simulink model "IMUControl"  (R2019b)
settings: Solver=FixedStepAuto  StartTime=0.0  StopTime=10.0  RelTol=1e-3
libraries: androidsensorlib x4, androiduilib x2, androidadvancedlib x1
settings Model: Creator=The MathWorks, Inc.  LastModifiedBy=Bilal
settings OptimizationCC: EnhancedBackFolding=on  PassReuseOutputArgsThreshold=0  MaxStackSize=64  OptimizeBlockOrder=speed  DifferentSizesBufferReuse=on  OptimizationCustomize=off
settings DebuggingCC: ParameterTunabilityLossMsg=error  ArithmeticOperatorsInVariantConditions=warning
settings HardwareCC: ProdBitPerPointer=32  ProdBitPerSizeT=32  ProdBitPerPtrDiffT=32  ProdLargestAtomicInteger=Long  ProdLargestAtomicFloat=Double  ProdWordSize=32  ProdHWDeviceType=ARM Compatible->ARM Cortex  UseEmbeddedCoderFeatures=off  UseSimulinkCoderFeatures=off
settings SFSimCC: MATLABDynamicMemAlloc=off  CustomCodeUndefinedFunction=UseInterfaceOnly
settings RTWCC: SystemTargetFile=ert.tlc  HardwareBoard=Android Device  TLCOptions="-aInlineSetEventsForThisBaseRateFcn=TLC_FALSE -aSuppressMultiTaskScheduler=TLC_FALSE  -aRateBasedStepFcn=0"  TemplateMakefile=ert_default_tmf  GenerateReport=on  RTWVerbose=off  Toolchain=Android SDK/NDK Tools  LaunchReport=on
settings CodeAppCC: ForceParamTrailComments=on  OperatorAnnotations=on
settings ERTTargetCC: ERTCustomFileBanners=off  SupportContinuousTime=on  SupportNonInlinedSFcns=on  RemoveResetFunc=off  ModelStepFunctionPrototypeControlCompliant=off

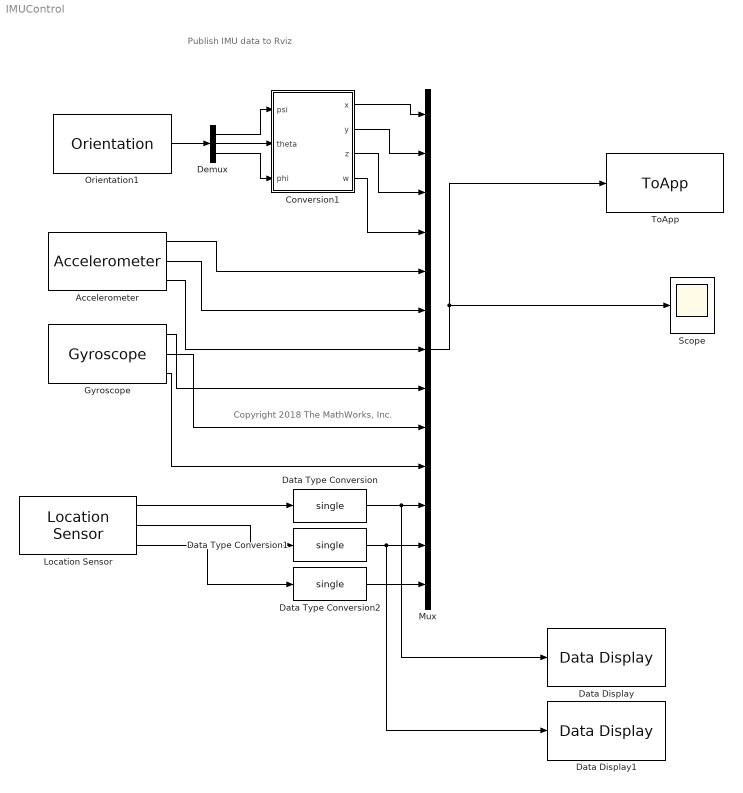
== system IMUControl ==
  note: Copyright 2018 The MathWorks, Inc.
  note: Publish IMU data to Rviz
  Accelerometer : androidsensorlib/Accelerometer  OutputVector=off  SampleTime=0.1  BlockPlatform=Android
      settings: SourceProductName=Simulink Support Package for Android Devices  SourceProductBaseCode=ANDROID
  Conversion1 : MATLAB Function  TreatAsAtomicUnit=on
  Data Display : androiduilib/Data Display  Format=Float  Precision=6  SimulateUsing=Code generation  blockPlatform=Android
      settings: SourceProductName=Simulink Support Package for Android Devices  SourceProductBaseCode=ANDROID
  Data Display1 : androiduilib/Data Display  Format=Float  Precision=6  SimulateUsing=Code generation  blockPlatform=Android
      settings: SourceProductName=Simulink Support Package for Android Devices  SourceProductBaseCode=ANDROID
  Data Type Conversion : DataTypeConversion  OutDataTypeStr=single
  Data Type Conversion1 : DataTypeConversion  OutDataTypeStr=single
  Data Type Conversion2 : DataTypeConversion  OutDataTypeStr=single
  Demux : Demux  Outputs=3
  Gyroscope : androidsensorlib/Gyroscope  OutputVector=off  SampleTime=0.1  BlockPlatform=Android
      settings: SourceProductName=Simulink Support Package for Android Devices  SourceProductBaseCode=ANDROID
  Location Sensor : androidsensorlib/Location Sensor  OutputVector=off  SampleTime=0.1  BlockPlatform=Android
      settings: SourceProductName=Simulink Support Package for Android Devices  SourceProductBaseCode=ANDROID
  Mux : Mux  Inputs=13
  Orientation1 : androidsensorlib/Orientation  SampleTime=0.1  SimulateUsing=Code generation
      settings: SourceProductName=Simulink Support Package for Android Devices  SourceProductBaseCode=ANDROID
  Scope : Scope
  ToApp : androidadvancedlib/ToApp  FunctionName=ROSPublish  NumInputs=1
      settings: SourceProductName=Simulink Support Package for Android Devices  SourceProductBaseCode=ANDROID
  wires:
  Gyroscope/1 -> Mux/8
  Conversion1/4(w) -> Mux/4
  Demux/2 -> Conversion1/2(theta)
  Accelerometer/2 -> Mux/6
  Accelerometer/3 -> Mux/7
  Conversion1/3(z) -> Mux/3
  Gyroscope/3 -> Mux/10
  Accelerometer/1 -> Mux/5
  Demux/1 -> Conversion1/1(psi)
  Mux/1 -> ToApp/1, Scope/1
  Orientation1/1 -> Demux/1
  Gyroscope/2 -> Mux/9
  Conversion1/2(y) -> Mux/2
  Demux/3 -> Conversion1/3(phi)
  Conversion1/1(x) -> Mux/1
  Location Sensor/1 -> Data Type Conversion/1
  Location Sensor/2 -> Data Type Conversion1/1
  Location Sensor/3 -> Data Type Conversion2/1
  Data Type Conversion/1 -> Data Display/1, Mux/11
  Data Type Conversion1/1 -> Data Display1/1, Mux/12
  Data Type Conversion2/1 -> Mux/13

== matlab function IMUControl/Conversion1 ==
  data: psi input; theta input; phi input; x output; y output; z output; w output
function  [x,y,z,w] = eul2quat(psi,theta,phi)
%#codegen

% Convert the quaternion to a yaw angle (zyx euler angle)
quat = eul2quat([phi,theta,psi]);
x = quat(1); y = quat(2); z = quat(3); w = quat(4);

end
